simulink model "AverageEEGStim"  (R2016b)
settings: Solver=FixedStepDiscrete  StartTime=0.0  StopTime=inf  FixedStep=sCoreParams.core.stepPeriod  RelTol=1e-3
undefined symbols (not defined in the file): sCoreParams
libraries: dspswit3 x1
settings Model: DataTypeOverride=Double  MinMaxOverflowLogging=ForceOff  Creator=anish  LastModifiedBy=Rina
settings SolverCC: EnableConcurrentExecution=on
settings DataIOCC: SaveFormat=StructureWithTime  SignalLoggingSaveFormat=ModelDataLogs  SaveOutput=off  SignalLogging=off  DSMLogging=off  SaveTime=off
settings OptimizationCC: BlockReduction=off  ConditionallyExecuteInputs=off  DefaultParameterBehavior=Inlined  OptimizeBlockIOStorage=off  BufferReuse=off  GlobalBufferReuse=off  ExpressionFolding=off  LocalBlockOutputs=off  LifeSpan=inf
settings DebuggingCC: SignalRangeChecking=error  SaveWithParameterizedLinksMsg=none  MultiTaskDSMMsg=warning  MultiTaskCondExecSysMsg=none  AllowSymbolicDim=off  ModelReferenceSymbolNameMessage=none  StateNameClashWarn=warning  SFUnexpectedBacktrackingDiag=warning  SFNoUnconditionalDefaultTransitionDiag=warning  SFExecutionAtInitializationDiag=none
settings HardwareCC: ProdBitPerPointer=32  ProdBitPerSizeT=32  ProdBitPerPtrDiffT=32  ProdLargestAtomicFloat=None  ProdWordSize=32  ProdLongLongMode=on  ProdHWDeviceType=Generic->32-bit x86 compatible  TargetBitPerPointer=64  TargetLargestAtomicFloat=Float  TargetLongLongMode=on  TargetIntDivRoundTo=Zero  TargetEndianess=LittleEndian  TargetWordSize=64  TargetHWDeviceType=Intel->x86-64 (Windows64)
settings ModelReferenceCC: UpdateModelReferenceTargets=Force  ModelReferencePassRootInputsByReference=off
settings RTWCC: SystemTargetFile=slrt.tlc  TemplateMakefile=slrt_default_tmf  Description=Simulink Real-Time  BuildConfiguration=Faster Runs  RTWCompilerOptimization=on
settings TargetCC: CodeReplacementLibrary=XPC_BLAS  ParMdlRefBuildCompliant=on  ConcurrentExecutionCompliant=on  GeneratePreprocessorConditionals=Use local settings  MatFileLogging=on  MATLABClassNameForMDSCustomization=xpcAperiodicCustomization
settings ConfigComp: CovMetricSettings=dw  CovHtmlReporting=on  CovSaveCumulativeToWorkspaceVar=on  CovSaveSingleToWorkspaceVar=on  CovExternalEMLEnable=off  CovSFcnEnable=off

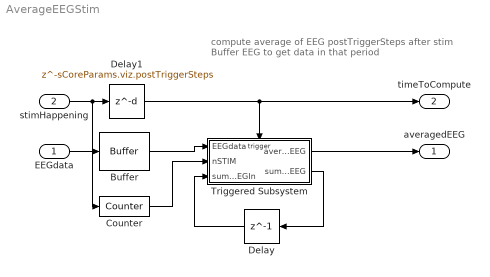
== system AverageEEGStim ==
  note: compute average of EEG  postTriggerSteps after stim
      | Buffer EEG to get data in that period
  EEGdata : Inport  PortDimensions=[sCoreParams.FrameSize sCoreParams.decoders.txDetector.nChannels]  SampleTime=sCoreParams.core.stepPeriod
  stimHappening : Inport  Port=2  OutDataTypeStr=boolean
  Buffer : Buffer  N=sCoreParams.viz.preTriggerSamp+sCoreParams.viz.postTriggerSamp  V=sCoreParams.viz.preTriggerSamp+sCoreParams.viz.postTriggerSamp-sCoreParams.FrameSize  TreatMby1Signals=One channel  OutputFrames=off
  Counter : dspswit3/Counter  Direction=Up  CountEvent=Rising edge  CounterSize=32 bits  MaxCount=2048  InitialCount=0  Output=Count  HitValue=32  ResetInput=off  SamplesPerFrame=1  Ts=1  CntDtype=double  HitDtype=Logical
  Delay : Delay  DelayLength=1
  Delay1 : Delay  DelayLength=sCoreParams.viz.postTriggerSteps
  Triggered Subsystem : Subsystem  TreatAsAtomicUnit=on
  averagedEEG : Outport  SampleTime=sCoreParams.core.stepPeriod
  timeToCompute : Outport  Port=2  SampleTime=sCoreParams.core.stepPeriod
  wires:
  EEGdata/1 -> Buffer/1
  Triggered Subsystem/1(averagedEEG) -> averagedEEG/1
  stimHappening/1 -> Counter/1, Delay1/1
  Delay/1 -> Triggered Subsystem/3(summedEEGIn)
  Delay1/1 -> timeToCompute/1, Triggered Subsystem/Trigger
  Buffer/1 -> Triggered Subsystem/1(EEGdata)
  Counter/1 -> Triggered Subsystem/2(nSTIM)
  Triggered Subsystem/2(summedEEG) -> Delay/1

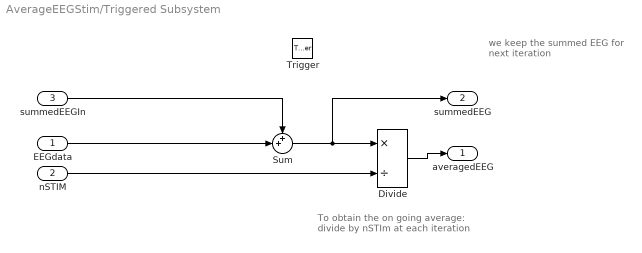
== system AverageEEGStim/Triggered Subsystem ==
  note: To obtain the on going average:
      | divide by nSTIm at each iteration
  note: we keep the summed EEG
      | for next iteration
  EEGdata : Inport
  nSTIM : Inport  Port=2
  summedEEGIn : Inport  Port=3
  Trigger : TriggerPort  VariantControl=Variant
  Divide : Product  Inputs=*/
  Sum : Sum  Inputs=++|
  averagedEEG : Outport
  summedEEG : Outport  Port=2
  wires:
  EEGdata/1 -> Sum/2
  Sum/1 -> summedEEG/1, Divide/1
  Divide/1 -> averagedEEG/1
  nSTIM/1 -> Divide/2
  summedEEGIn/1 -> Sum/1
